simulink model "lab2_2"  (R2022a)
settings: Solver=VariableStepAuto  StartTime=0.0  StopTime=10.0  RelTol=1e-3
settings Model: Creator=HP  LastModifiedBy=HP

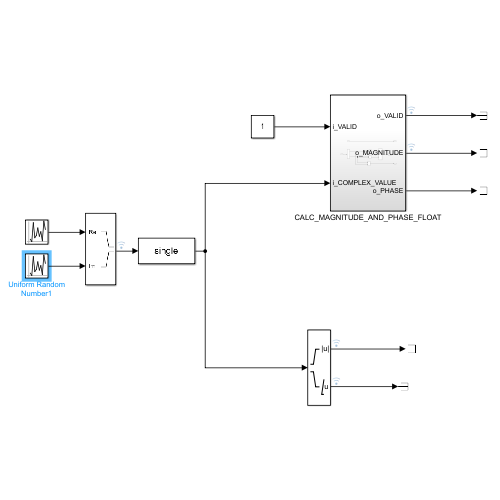
[thumbnail: Simulink's stored preview of the top-level diagram]
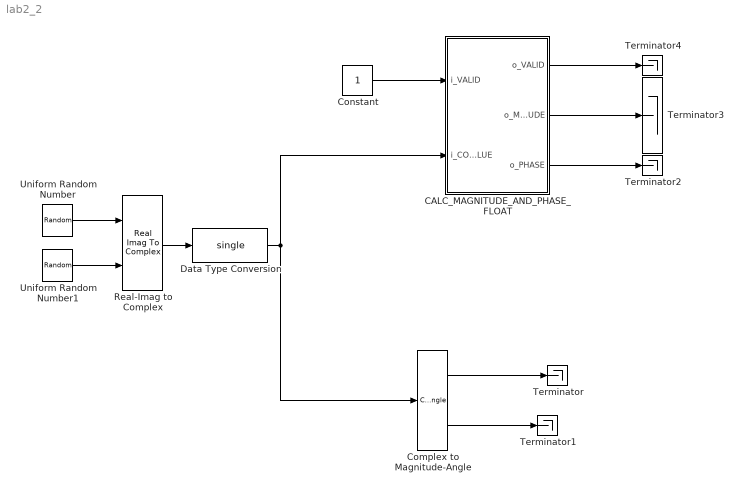
== system lab2_2 ==
  CALC_MAGNITUDE_AND_PHASE_FLOAT : Subsystem
  Complex to Magnitude-Angle : ComplexToMagnitudeAngle
  Constant : Constant  OutDataTypeStr=boolean  SampleTime=1
  Data Type Conversion : DataTypeConversion  OutDataTypeStr=single  SaturateOnIntegerOverflow=off  RndMeth=Floor
  Real-Imag to Complex : RealImagToComplex
  Terminator{,1..4} (5 alike) : Terminator
  Uniform Random Number : UniformRandomNumber  Minimum=0  Maximum=1.99999999953433871269  Seed=1  SampleTime=1
  Uniform Random Number1 : UniformRandomNumber  Minimum=0  Maximum=1.99999999953433871269  Seed=2  SampleTime=1
  wires:
  Complex to Magnitude-Angle/2 -> Terminator1/1
  Data Type Conversion/1 -> Complex to Magnitude-Angle/1, CALC_MAGNITUDE_AND_PHASE_FLOAT/2(i_COMPLEX_VALUE)
  Constant/1 -> CALC_MAGNITUDE_AND_PHASE_FLOAT/1(i_VALID)
  Uniform Random Number1/1 -> Real-Imag to Complex/2
  Real-Imag to Complex/1 -> Data Type Conversion/1
  Complex to Magnitude-Angle/1 -> Terminator/1
  Uniform Random Number/1 -> Real-Imag to Complex/1
  CALC_MAGNITUDE_AND_PHASE_FLOAT/3(o_PHASE) -> Terminator2/1
  CALC_MAGNITUDE_AND_PHASE_FLOAT/2(o_MAGNITUDE) -> Terminator3/1
  CALC_MAGNITUDE_AND_PHASE_FLOAT/1(o_VALID) -> Terminator4/1

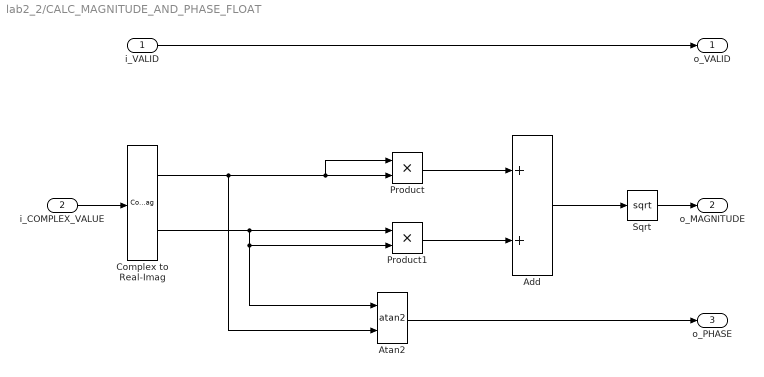
== system lab2_2/CALC_MAGNITUDE_AND_PHASE_FLOAT ==
  i_VALID : Inport  OutDataTypeStr=boolean
  i_COMPLEX_VALUE : Inport  Port=2  OutDataTypeStr=single
  Add : Sum  OutDataTypeStr=single
  Atan2 : Trigonometry  Operator=atan2  NumberOfIterations=20
  Complex to Real-Imag : ComplexToRealImag
  Product : Product  OutDataTypeStr=single  SaturateOnIntegerOverflow=on
  Product1 : Product  OutDataTypeStr=single  LockScale=on
  Sqrt : Sqrt  OutDataTypeStr=single
  o_VALID : Outport  OutDataTypeStr=boolean
  o_MAGNITUDE : Outport  Port=2  OutDataTypeStr=single
  o_PHASE : Outport  Port=3  OutDataTypeStr=single
  wires:
  Complex to Real-Imag/2 -> Product1/1, Atan2/1, Product1/2
  Complex to Real-Imag/1 -> Atan2/2, Product/1, Product/2
  Atan2/1 -> o_PHASE/1
  Product1/1 -> Add/2
  Product/1 -> Add/1
  Add/1 -> Sqrt/1
  i_VALID/1 -> o_VALID/1
  i_COMPLEX_VALUE/1 -> Complex to Real-Imag/1
  Sqrt/1 -> o_MAGNITUDE/1
